simulink model "VELOCITY_MODEL"  (R2014b)
settings: Solver=ode45  StartTime=0.0  StopTime=30  RelTol=1e-3
libraries: simulink x2
settings Model: Creator=a_botros  LastModifiedBy=a_botros
settings DebuggingCC: UnderspecifiedInitializationDetection=Classic  MergeDetectMultiDrivingBlocksExec=none  StateNameClashWarn=warning

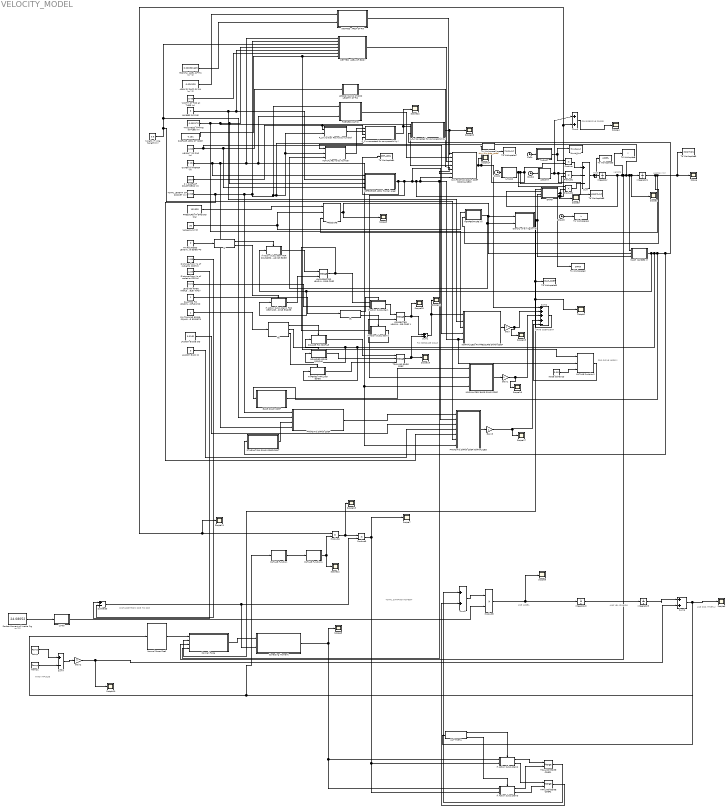
== system VELOCITY_MODEL ==
  note: FOR OGIVE NOSE!!!
  note: WIND IMPULSE
  note: ANG POS (THETA)
  note: ANG VEL (OMEGA)
  note: ANG ACCEL
  note: TOTAL DAMPING MOMENT
  note: DISTANCE FROM COG TO COP
  note: COMPRESSIVE
      | FORCE
  note: DRAG COEFICIENT
  note: FIN PRESSURE DRAG
  note: position (m)
  note: velocity
  note: accel
  1/MASS : MATLAB Function  TreatAsAtomicUnit=on
  1/MOI : MATLAB Function  TreatAsAtomicUnit=on
  ACTUAL Reynolds Number : MATLAB Function  TreatAsAtomicUnit=on
  AERODYNAMIC CHORD LENGTH OF FIN : MATLAB Function  TreatAsAtomicUnit=on
  AREA OF FACE OF FIN (m^2) : Constant  Value=0.026125
  BASE DRAG COEF : MATLAB Function  TreatAsAtomicUnit=on
  CORRECTED LEADING EDGE COEF 1 : Merge
  C_f (uncorrected for compressibility) : MATLAB Function  TreatAsAtomicUnit=on
  C_f_c (corrected for compressibility) : MATLAB Function  TreatAsAtomicUnit=on
  Clock{,1..3} (4 alike) : Clock
  Correcting Moment : MATLAB Function  TreatAsAtomicUnit=on
  DRAG : MATLAB Function  TreatAsAtomicUnit=on
  Density of air (kg/m^3) : MATLAB Function  TreatAsAtomicUnit=on
  Distance from tip of rocket to COG(m) : Constant  Value=1.88
  Distance from tip of rocket to COP(m) : Constant  Value=2.05
  FIN ROUNDED LEADING EDGE=1 RECT' LEADING EDGE =0 : Constant  Value=0
  "FIN TRAILING EDGE: SQUARE FIN PROFILE=1 ROUNDED EDGE PROFILE=2 TAPERED TRAILING EDGE=3 " : Constant
  FINENESS RATIO : MATLAB Function  TreatAsAtomicUnit=on
  FRONTAL AREA OF FIN (m^2) : Constant  Value=0.000301625
  Gain : Gain
  Gain1 : Gain
  Gain2 : Gain  Gain=0
  Gain3 : Gain
  HEIGHT OF FINS (m) : Constant  Value=0.95
  If : If  IfExpression=u1==1
  If Action Subsystem : Subsystem  TreatAsAtomicUnit=on
  If Action Subsystem FOR ROUNDED LEADING EDGE : Subsystem  TreatAsAtomicUnit=on
  If Action Subsystem1 : Subsystem  TreatAsAtomicUnit=on
  If Action Subsystem1 FOR RECTANGULAR LEADING ENDGE : Subsystem  TreatAsAtomicUnit=on
  If Action Subsystem2 : Subsystem  TreatAsAtomicUnit=on
  If Action Subsystem3 : Subsystem  TreatAsAtomicUnit=on
  If1 : If  IfExpression=u1 == 1
  If2 : If  IfExpression=u1 ==1  ElseIfExpressions=u1==2
  Integrator{,1..3} (4 alike) : Integrator
  LAUNCH GUID ID : Constant  Value=0
  LAUNCH GUIDE OD : Constant  Value=0.0161
  LEADING EDGE ANGLE (IF APPLICABLE) (RAD) : Constant  Value=0.21
  MACH NUMBER M : MATLAB Function  TreatAsAtomicUnit=on
  MATLAB Function : MATLAB Function  TreatAsAtomicUnit=on
  MATLAB Function1 : MATLAB Function  TreatAsAtomicUnit=on
  MATLAB Function2 : MATLAB Function  TreatAsAtomicUnit=on
  NORMALIZED BASE DRAG COEF : MATLAB Function  TreatAsAtomicUnit=on
  NORMALIZED FIN PRESSURE DRAG COEF : MATLAB Function  TreatAsAtomicUnit=on
  NOSE CONE CD : Constant  Value=0.05
  NUMBER OF FINS : Constant  Value=3
  Normal Force : MATLAB Function  TreatAsAtomicUnit=on
  Normal Force Coef : MATLAB Function  TreatAsAtomicUnit=on
  OUTER DIAMETER (m) : Constant  Value=0.104
  PARASITIC DRAG COEF : MATLAB Function  TreatAsAtomicUnit=on
  PARASITIC DRAG COEF NORMALIZED : MATLAB Function  TreatAsAtomicUnit=on
  PRESSURE : MATLAB Function  TreatAsAtomicUnit=on
  PRESSURE AT GROUND (Pa) : Constant  Value=101325
  Product{,1..5} (6 alike) : Product
  REFERENCE AREA (frontal area) : MATLAB Function  TreatAsAtomicUnit=on
  ROUNDED EDGE PROFILE : Subsystem  TreatAsAtomicUnit=on
  R_crit (critical Reynolds number) : MATLAB Function  TreatAsAtomicUnit=on
  R_s SURFACE ROUGHNESS (m) : Constant  Value=20E-6
  Ramp : simulink/Sources/Ramp  slope=5  start=2  X0=0
  Ramp1 : simulink/Sources/Ramp  slope=-5  start=2.0001  X0=0
  Rocket Moment of Inertia (kg m^2) : Constant  Value=24.08052
  SKN FRICTION DRAG COEF (NORMALIZED) : MATLAB Function  TreatAsAtomicUnit=on
  SLANTED FIN LEADING EDGE=1 FIN PERPENDICULAR TO AIRFLOW=0 : Constant
  SQUARE FIN PROFILE : Subsystem  TreatAsAtomicUnit=on
  STAGNATION DRAG COEFICIENT : MATLAB Function  TreatAsAtomicUnit=on
  SURFACE AREA OF NOSE : Constant  Value=0.131
  Scope{,1..22} (23 alike) : Scope
      Scope10 settings: SaveName=ScopeData10
      Scope11 settings: SaveName=ScopeData11
      Scope12 settings: SaveName=ScopeData12
      Scope13 settings: SaveName=ScopeData13
      Scope14 settings: SaveName=ScopeData14
      Scope15 settings: SaveName=ScopeData15
      Scope16 settings: SaveName=ScopeData16
      Scope17 settings: SaveName=ScopeData17
      Scope18 settings: SaveName=ScopeData18
      Scope19 settings: SaveName=ScopeData19
      Scope2 settings: SaveName=ScopeData2
      Scope20 settings: SaveName=ScopeData20
      Scope21 settings: SaveName=ScopeData21
      Scope22 settings: SaveName=ScopeData22
      Scope3 settings: SaveName=ScopeData3
      Scope4 settings: SaveName=ScopeData4
      Scope5 settings: SaveName=ScopeData5
      Scope6 settings: YMin=25000  YMax=105000  SaveName=ScopeData6
      Scope7 settings: SaveName=ScopeData7
      Scope8 settings: SaveName=ScopeData8
      Scope9 settings: SaveName=ScopeData9
  Subtract3 : Sum  Inputs=+-
  Sum : Sum  Inputs=+--
  Sum1 : Sum
  Sum2 : Sum  Inputs=++++-
  Sum3 : Sum  Inputs=|++
  Sum5 : Sum
  Sum6 : Sum  Inputs=|++
  Sum7 : Sum  Inputs=+-
  TAPERED TRAILING EDGE : Subsystem  TreatAsAtomicUnit=on
  TEMPERATURE (K) : MATLAB Function  TreatAsAtomicUnit=on
  THICKNESS OF FINS at TUBE (m) : Constant  Value=0.003175
  THRUST : MATLAB Function  TreatAsAtomicUnit=on
  TOTAL LENGTH OF ROCKET (m) : Constant  Value=2.98
  TRAILING EDGE COEF : Merge  Inputs=3
  TRAILING EDGE COEF1 : Merge
  TRAILING EDGE COEF2 : Merge
  To Workspace : ToWorkspace  VariableName=v  SampleTime=-1
  To Workspace1 : ToWorkspace  VariableName=t  SampleTime=-1
  To Workspace2 : ToWorkspace  VariableName=DRAG  SampleTime=-1
  To Workspace3 : ToWorkspace  VariableName=ACCEL  SaveFormat=Timeseries  SampleTime=-1
  To Workspace4 : ToWorkspace  VariableName=REF_AREA  SampleTime=-1
  To Workspace5 : ToWorkspace  VariableName=POSITION  SampleTime=-1
  To Workspace6 : ToWorkspace  VariableName=DRAG_COEF  SampleTime=-1
  To Workspace7 : ToWorkspace  VariableName=mass_out  SampleTime=-1
  To Workspace8 : ToWorkspace  VariableName=weight_out  SampleTime=-1
  To Workspace9 : ToWorkspace  VariableName=skin_fric_drag_cofef  SampleTime=-1
  U1+THETA : If
  "UNCORRECTED LEADING EDGE COEF " : Merge
  WEIGHT : MATLAB Function  TreatAsAtomicUnit=on
  WETTED  AREA OF BODY : MATLAB Function  TreatAsAtomicUnit=on
  WETTED  AREA OF FIN : MATLAB Function  TreatAsAtomicUnit=on
  WIDTH OF FINS at TUBE (m) : Constant  Value=0.45
  height of nose (length)(m) : Constant  Value=0.6
  t_at_ground (C) : Constant  Value=30
  "thrust_out " : ToWorkspace  VariableName=thrust_out  SampleTime=-1
  wires:
  THRUST/1(T) -> "thrust_out "/1, Product/1
  1/MASS/1(M) -> Product2/1, Product1/2, Product/2, To Workspace7/1
  Clock/1 -> THRUST/1(t)
  Clock1/1 -> 1/MASS/1(t)
  Product/1 -> Sum/1
  Clock2/1 -> WEIGHT/1(t)
  Product1/1 -> Sum/2
  DRAG/1(D) -> To Workspace2/1, Scope3/1, Scope11/1, Product4/1, Sum3/2, Product2/2
  Product2/1 -> Sum/3
  Integrator/1 -> DRAG/2(v), Normal Force/3(v), ACTUAL Reynolds Number/1(v), MACH NUMBER M/1(v), Scope1/1, Integrator1/1, To Workspace/1
  Sum/1 -> To Workspace3/1, Integrator/1
  WEIGHT/1(W) -> Sum3/1, To Workspace8/1, Product1/1
  Clock3/1 -> To Workspace1/1
  Integrator1/1 -> PRESSURE/3(x), To Workspace5/1, Scope/1, TEMPERATURE (K)/2(x)
  Density of air (kg/m^3)/1(ro) -> Normal Force/2(ro), DRAG/3(ro), MACH NUMBER M/3(ro)
  TEMPERATURE (K)/1(T) -> ACTUAL Reynolds Number/3(T), Density of air (kg/m^3)/2(T)
  t_at_ground (C)/1 -> TEMPERATURE (K)/1(t_at_ground), PRESSURE/2(t_0)
  PRESSURE/1(p) -> Density of air (kg/m^3)/1(p), MACH NUMBER M/2(p), Scope5/1
  R_s SURFACE ROUGHNESS (m)/1 -> C_f (uncorrected for compressibility)/3(R_s), R_crit (critical Reynolds number)/1(R_s)
  TOTAL LENGTH OF ROCKET (m)/1 -> PARASITIC DRAG COEF NORMALIZED/5(L), PARASITIC DRAG COEF/1(L), FINENESS RATIO/1(L), C_f (uncorrected for compressibility)/4(L), R_crit (critical Reynolds number)/2(L), ACTUAL Reynolds Number/2(L), WETTED  AREA OF BODY/2(L)
  ACTUAL Reynolds Number/1(R) -> C_f (uncorrected for compressibility)/1(R)
  R_crit (critical Reynolds number)/1(R_crit) -> C_f (uncorrected for compressibility)/2(R_crit)
  C_f (uncorrected for compressibility)/1(C_f) -> Scope22/1, C_f_c (corrected for compressibility)/1(C_f)
  MACH NUMBER M/1(M) -> If Action Subsystem1 FOR RECTANGULAR LEADING ENDGE/1(In1), If Action Subsystem FOR ROUNDED LEADING EDGE/1(In1), TAPERED TRAILING EDGE/1(In1), ROUNDED EDGE PROFILE/1(In1), SQUARE FIN PROFILE/1(In1), BASE DRAG COEF/1(M), STAGNATION DRAG COEFICIENT/1(M), C_f_c (corrected for compressibility)/2(M)
  PRESSURE AT GROUND (Pa)/1 -> PRESSURE/1(p_0)
  OUTER DIAMETER (m)/1 -> PARASITIC DRAG COEF NORMALIZED/7(OD), NORMALIZED BASE DRAG COEF/3(OD), FINENESS RATIO/2(OD), WETTED  AREA OF BODY/1(OD), PARASITIC DRAG COEF/4(OD), REFERENCE AREA (frontal area)/1(OD)
  HEIGHT OF FINS (m)/1 -> NORMALIZED FIN PRESSURE DRAG COEF/4(s), REFERENCE AREA (frontal area)/4(s), AERODYNAMIC CHORD LENGTH OF FIN/1(s)
  height of nose (length)(m)/1 -> PARASITIC DRAG COEF NORMALIZED/6(h), PARASITIC DRAG COEF/2(h), WETTED  AREA OF BODY/3(h)
  SURFACE AREA OF NOSE/1 -> WETTED  AREA OF BODY/7(A_surface_nose), MATLAB Function2/1(A)
  THICKNESS OF FINS at TUBE (m)/1 -> NORMALIZED FIN PRESSURE DRAG COEF/3(t), SKN FRICTION DRAG COEF (NORMALIZED)/4(t), REFERENCE AREA (frontal area)/3(t), WETTED  AREA OF BODY/4(t)
  NUMBER OF FINS/1 -> REFERENCE AREA (frontal area)/2(N), WETTED  AREA OF BODY/5(N), NORMALIZED FIN PRESSURE DRAG COEF/2(N)
  WIDTH OF FINS at TUBE (m)/1 -> WETTED  AREA OF BODY/6(l)
  FRONTAL AREA OF FIN (m^2)/1 -> WETTED  AREA OF FIN/2(A_front_fin)
  AREA OF FACE OF FIN (m^2)/1 -> WETTED  AREA OF FIN/1(A_face_fin)
  STAGNATION DRAG COEFICIENT/1(C_stag) -> PARASITIC DRAG COEF/3(C_stag)
  FIN ROUNDED LEADING EDGE=1 RECT' LEADING EDGE =0/1 -> If/1
  If/1 -> If Action Subsystem FOR ROUNDED LEADING EDGE/Action
  If/2 -> If Action Subsystem1 FOR RECTANGULAR LEADING ENDGE/Action
  If Action Subsystem FOR ROUNDED LEADING EDGE/1(Out1) -> "UNCORRECTED LEADING EDGE COEF "/1
  If Action Subsystem1 FOR RECTANGULAR LEADING ENDGE/1(Out1) -> "UNCORRECTED LEADING EDGE COEF "/2
  SLANTED FIN LEADING EDGE=1 FIN PERPENDICULAR TO AIRFLOW=0/1 -> If1/1
  If1/2 -> If Action Subsystem1/Action
  If1/1 -> If Action Subsystem/Action
  "UNCORRECTED LEADING EDGE COEF "/1 -> If Action Subsystem1/1(In1), If Action Subsystem/1(In1)
  LEADING EDGE ANGLE (IF APPLICABLE) (RAD)/1 -> If Action Subsystem/2(In2)
  If Action Subsystem/1(Out1) -> CORRECTED LEADING EDGE COEF 1/1
  If Action Subsystem1/1(Out1) -> CORRECTED LEADING EDGE COEF 1/2
  "FIN TRAILING EDGE: SQUARE FIN PROFILE=1 ROUNDED EDGE PROFILE=2 TAPERED TRAILING EDGE=3 "/1 -> If2/1
  If2/1 -> SQUARE FIN PROFILE/Action
  If2/2 -> ROUNDED EDGE PROFILE/Action
  If2/3 -> TAPERED TRAILING EDGE/Action
  SQUARE FIN PROFILE/1(Out1) -> TRAILING EDGE COEF/1
  ROUNDED EDGE PROFILE/1(Out1) -> TRAILING EDGE COEF/2
  TAPERED TRAILING EDGE/1(Out1) -> TRAILING EDGE COEF/3
  CORRECTED LEADING EDGE COEF 1/1 -> Scope18/1, Sum1/1
  C_f_c (corrected for compressibility)/1(C_f_c) -> Scope20/1, SKN FRICTION DRAG COEF (NORMALIZED)/1(C_f_c)
  FINENESS RATIO/1(f_b) -> SKN FRICTION DRAG COEF (NORMALIZED)/2(f_b)
  WETTED  AREA OF BODY/1(A_wet_body) -> SKN FRICTION DRAG COEF (NORMALIZED)/3(A_wet_body)
  AERODYNAMIC CHORD LENGTH OF FIN/1(c) -> SKN FRICTION DRAG COEF (NORMALIZED)/5(c)
  WETTED  AREA OF FIN/1(A_wet_fin) -> SKN FRICTION DRAG COEF (NORMALIZED)/6(A_wet_fins)
  REFERENCE AREA (frontal area)/1(A_ref) -> To Workspace4/1, Normal Force/4(A_ref), MATLAB Function2/2(A_ref), NORMALIZED FIN PRESSURE DRAG COEF/5(A_ref), SKN FRICTION DRAG COEF (NORMALIZED)/7(A_ref), DRAG/4(A_ref), PARASITIC DRAG COEF NORMALIZED/2(A_ref), NORMALIZED BASE DRAG COEF/2(A_ref)
  Sum1/1 -> Scope21/1, NORMALIZED FIN PRESSURE DRAG COEF/1(fin_pressure_drag)
  BASE DRAG COEF/1(C_base) -> NORMALIZED BASE DRAG COEF/1(C_base)
  PARASITIC DRAG COEF/1(C_parasitic) -> PARASITIC DRAG COEF NORMALIZED/1(C_parasitic)
  LAUNCH GUIDE OD/1 -> PARASITIC DRAG COEF NORMALIZED/3(r_ext)
  LAUNCH GUID ID/1 -> PARASITIC DRAG COEF NORMALIZED/4(r_int)
  TRAILING EDGE COEF/1 -> Scope19/1, Sum1/2
  SKN FRICTION DRAG COEF (NORMALIZED)/1(C_D_fric) -> Scope14/1, To Workspace9/1, Sum2/1
  Gain/1 -> Scope15/1, Sum2/2
  Gain1/1 -> Scope16/1, Sum2/3
  Gain3/1 -> Sum2/4, Scope17/1
  Sum2/1 -> Scope2/1, DRAG/1(Cd), To Workspace6/1
  Sum3/1 -> Scope4/1
  Distance from tip of rocket to COG(m)/1 -> Subtract3/2
  Distance from tip of rocket to COP(m)/1 -> Subtract3/1
  Subtract3/1 -> Product5/2, Correcting Moment/2(d_t)
  Normal Force Coef/1(C_N) -> Normal Force/1(C_N)
  Normal Force/1(N) -> Correcting Moment/1(N)
  Correcting Moment/1(M_correcting) -> If Action Subsystem3/1(N), If Action Subsystem2/1(N), Scope8/1
  Sum5/1 -> Product3/1
  Rocket Moment of Inertia (kg m^2)/1 -> 1/MOI/1(u)
  1/MOI/1(y) -> Product3/2
  Product3/1 -> Scope9/1, Integrator2/1
  Integrator2/1 -> Integrator3/1
  Gain2/1 -> Scope10/1, Sum6/2
  Integrator3/1 -> Sum6/1
  Sum6/1 -> U1+THETA/1, Scope6/1, MATLAB Function/1(deg), Normal Force Coef/1(theta)
  Ramp/1 -> Sum7/1
  Ramp1/1 -> Sum7/2
  Sum7/1 -> Gain2/1
  MATLAB Function/1(rad) -> MATLAB Function1/1(u)
  MATLAB Function1/1(y) -> Product4/2, Scope12/1
  Product4/1 -> Scope13/1, Product5/1
  Product5/1 -> If Action Subsystem3/2(D), If Action Subsystem2/2(D), Scope7/1
  U1+THETA/1 -> If Action Subsystem2/Action
  U1+THETA/2 -> If Action Subsystem3/Action
  If Action Subsystem2/1(Nout) -> TRAILING EDGE COEF1/1
  If Action Subsystem3/1(Nout) -> TRAILING EDGE COEF1/2
  If Action Subsystem3/2(Dout) -> TRAILING EDGE COEF2/2
  If Action Subsystem2/2(Dout) -> TRAILING EDGE COEF2/1
  TRAILING EDGE COEF1/1 -> Sum5/1
  TRAILING EDGE COEF2/1 -> Sum5/2
  NORMALIZED FIN PRESSURE DRAG COEF/1(C_D_pressure) -> Gain/1
  NORMALIZED BASE DRAG COEF/1(C_base_n) -> Gain1/1
  PARASITIC DRAG COEF NORMALIZED/1(C_parasitic_norm) -> Gain3/1
  NOSE CONE CD/1 -> MATLAB Function2/3(CND)
  MATLAB Function2/1(y) -> Sum2/5

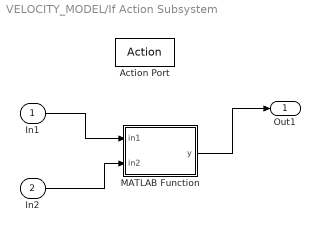
== system VELOCITY_MODEL/If Action Subsystem ==
  In1 : Inport
  In2 : Inport  Port=2
  Action Port : ActionPort  ActionType=then
  MATLAB Function : MATLAB Function  TreatAsAtomicUnit=on
  Out1 : Outport
  wires:
  In1/1 -> MATLAB Function/1(in1)
  In2/1 -> MATLAB Function/2(in2)
  MATLAB Function/1(y) -> Out1/1

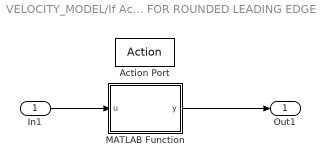
== system VELOCITY_MODEL/If Action Subsystem FOR ROUNDED LEADING EDGE ==
  In1 : Inport
  Action Port : ActionPort  ActionType=then
  MATLAB Function : MATLAB Function  TreatAsAtomicUnit=on
  Out1 : Outport
  wires:
  In1/1 -> MATLAB Function/1(u)
  MATLAB Function/1(y) -> Out1/1

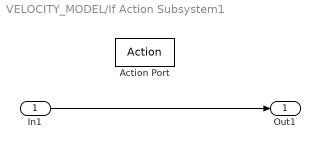
== system VELOCITY_MODEL/If Action Subsystem1 ==
  In1 : Inport
  Action Port : ActionPort  ActionType=else
  Out1 : Outport
  wires:
  In1/1 -> Out1/1

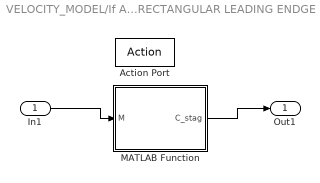
== system VELOCITY_MODEL/If Action Subsystem1 FOR RECTANGULAR LEADING ENDGE ==
  In1 : Inport
  Action Port : ActionPort  ActionType=else
  MATLAB Function : MATLAB Function  TreatAsAtomicUnit=on
  Out1 : Outport
  wires:
  In1/1 -> MATLAB Function/1(M)
  MATLAB Function/1(C_stag) -> Out1/1

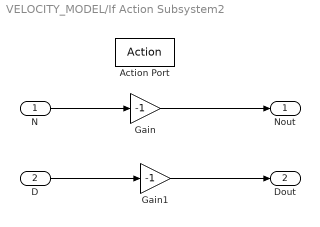
== system VELOCITY_MODEL/If Action Subsystem2 ==
  N : Inport
  D : Inport  Port=2
  Action Port : ActionPort  ActionType=then
  Gain : Gain  Gain=-1
  Gain1 : Gain  Gain=-1
  Nout : Outport
  Dout : Outport  Port=2
  wires:
  N/1 -> Gain/1
  Gain/1 -> Nout/1
  D/1 -> Gain1/1
  Gain1/1 -> Dout/1

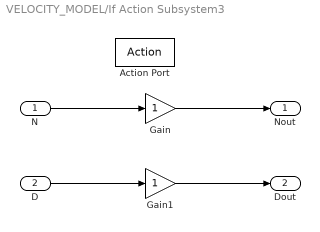
== system VELOCITY_MODEL/If Action Subsystem3 ==
  N : Inport
  D : Inport  Port=2
  Action Port : ActionPort  ActionType=else
  Gain : Gain
  Gain1 : Gain
  Nout : Outport
  Dout : Outport  Port=2
  wires:
  N/1 -> Gain/1
  Gain/1 -> Nout/1
  D/1 -> Gain1/1
  Gain1/1 -> Dout/1

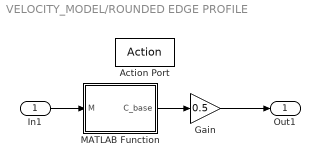
== system VELOCITY_MODEL/ROUNDED EDGE PROFILE ==
  In1 : Inport
  Action Port : ActionPort  ActionType=elseif
  Gain : Gain  Gain=0.5
  MATLAB Function : MATLAB Function  TreatAsAtomicUnit=on
  Out1 : Outport
  wires:
  In1/1 -> MATLAB Function/1(M)
  MATLAB Function/1(C_base) -> Gain/1
  Gain/1 -> Out1/1

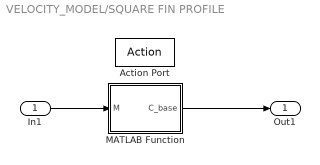
== system VELOCITY_MODEL/SQUARE FIN PROFILE ==
  In1 : Inport
  Action Port : ActionPort  ActionType=then
  MATLAB Function : MATLAB Function  TreatAsAtomicUnit=on
  Out1 : Outport
  wires:
  In1/1 -> MATLAB Function/1(M)
  MATLAB Function/1(C_base) -> Out1/1

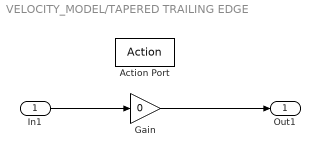
== system VELOCITY_MODEL/TAPERED TRAILING EDGE ==
  In1 : Inport
  Action Port : ActionPort  ActionType=else
  Gain : Gain  Gain=0
  Out1 : Outport
  wires:
  In1/1 -> Gain/1
  Gain/1 -> Out1/1

== matlab function VELOCITY_MODEL/WEIGHT ==
  data: t input; W output
function W   = WEIGHT( t )
if t<=4.7012
    W=(75.94*t^2-1234.5*t+20937)/1000*9.80665 

else
    W=17092/1000*9.80665 
end


end

== matlab function VELOCITY_MODEL/THRUST ==
  data: t input; T output
function  T  = THRUST(t)
%YIELDS THRUST CURVE OVER TIME
if t<0.08
    T=4000000*t^3-462933*t^2+41915*t+209.66
elseif t<0.15935
    T=-4701*t+2748.7
elseif t<0.21276 
    T=-1133.2*t+2223.6 
elseif t<0.32775
    T=787.15*t+1850.2
elseif t<0.57775
    T=-754.4*t+2339.9  
elseif t<0.72775
    T=-251*t+2070.7 
elseif t<1.7277
    T=-70.147*t+1947.4
elseif t<3.3777
    T=-31.421*t^2-9.1503*t+1930.8
elseif t<3.9777
    T=3656.6*t^3-39167*t^2+137806*t-158018
elseif t<4.5277
    T=-1051.8*t+4709.4
else
    T=0
    
      
   end


end

== matlab function VELOCITY_MODEL/1//MASS ==
  data: t input; M output
function M   = MASSRECIP( t )

if t<=4.7012
    M=1/((75.94*t^2-1234.5*t+20937)/1000)

else
    M=1/(17092/1000) 
end

end

== matlab function VELOCITY_MODEL/DRAG ==
  data: Cd input; D output; v input; ro input; A_ref input
function D = DRAG(Cd, v, ro, A_ref)
%#codegen
D=0.5*Cd*v^2*A_ref*ro
end

== matlab function VELOCITY_MODEL/NORMALIZED FIN PRESSURE DRAG COEF ==
  data: fin_pressure_drag input; C_D_pressure output; N input; t input; s input; A_ref input
function C_D_pressure = PRESS(fin_pressure_drag, N ,t ,s, A_ref)
%#codegen

C_D_pressure = fin_pressure_drag*N*t*s/A_ref;
end

== matlab function VELOCITY_MODEL/Density of air (kg//m^3) ==
  data: p input; ro output; T input
function ro = DENSITYOFAIR(p,T)
%#codegen
ro=p*0.0289644/(8.31447*T)
end

== matlab function VELOCITY_MODEL/TEMPERATURE (K) ==
  data: t_at_ground input; T output; x input
function T = t(t_at_ground, x)
%#codegen
double m;
if x<11000
    m=-6.5
elseif x<11019
    m=0
else 
    m=1
end
    
    
    
    
    
T=(t_at_ground+274.15-m/1000*x)
end

== matlab function VELOCITY_MODEL/If Action Subsystem/MATLAB Function ==
  data: in1 input; y output; in2 input
function y = fcn(in1, in2)
%#codegen
y=in1*cos(in2)^2
end

== matlab function VELOCITY_MODEL/REFERENCE AREA (frontal area) ==
  data: OD input; A_ref output; N input; t input; s input
function A_ref = REFAREA(OD, N, t, s)
%#codegen

%A_ref=3.14159*OD^2/4+t*s*N
A_ref=0.0084949
end

== matlab function VELOCITY_MODEL/BASE DRAG COEF ==
  data: M input; C_base output
function C_base = BASEDRAG(M)
%#codegen
if M<1
    C_base=0.12+0.13*M^2
else
    C_base=0.25/M
end

end

== matlab function VELOCITY_MODEL/PARASITIC DRAG COEF ==
  data: L input; C_parasitic output; h input; C_stag input; OD input
function C_parasitic = PARASITICDRAG(L,h,C_stag,OD)
%#codegen
C_parasitic=max(1.3-0.3*(L-h)/OD, 1)*C_stag
end

== matlab function VELOCITY_MODEL/R_crit (critical Reynolds number) ==
  data: R_s input; R_crit output; L input
function R_crit = CRITREN(R_s, L)
%#codegen

R_crit=51*(R_s/L)^(-1.039);
end

== matlab function VELOCITY_MODEL/C_f (uncorrected for compressibility) ==
  data: R input; C_f output; R_crit input; R_s input; L input
function C_f = SKNDRAGCOEF(R, R_crit, R_s, L)
%#codegen
if R<1E4
  C_f=0.0148
elseif R<R_crit
  C_f=1/(1.5*log(R)-5.6)^2 
else
  C_f=0.032*(R_s/L)^(0.2)
end 


end

== matlab function VELOCITY_MODEL/ACTUAL Reynolds Number ==
  data: v input; R output; L input; T input
function R = ACTREN(v, L, T)
%#codegen

R=v*L/(-1E-14*T^3+1E-10*T^2+3E-8*T-3E-6);
end

== matlab function VELOCITY_MODEL/MACH NUMBER M ==
  data: v input; M output; p input; ro input
function M = MACH(v, p, ro)
%#codegen

M=v/sqrt(1.4*p/ro)
end

== matlab function VELOCITY_MODEL/C_f_c (corrected for compressibility) ==
  data: C_f input; C_f_c output; M input
function C_f_c = SKNDRAGCOEFCORR(C_f, M)
%#codegen
double CC;
CC=C_f*(1-0.1*M^2);

if CC>C_f
  C_f_c=CC
else
  C_f_c=C_f
end

end

== matlab function VELOCITY_MODEL/PRESSURE ==
  data: p_0 input; p output; t_0 input; x input
function p = PRESSURE(p_0, t_0, x)
%#codegen
p=p_0*(1-0.0065*x/(t_0+274.15))^(9.80665*0.0289644/(8.31447*0.0065))
end

== matlab function VELOCITY_MODEL/FINENESS RATIO ==
  data: L input; f_b output; OD input
function f_b = FINENESS(L, OD)
%#codegen

f_b=L/OD
end

== matlab function VELOCITY_MODEL/AERODYNAMIC CHORD LENGTH OF FIN ==
  data: s input; c output
function c = ACL(s)
%#codegen
c=s
end

== matlab function VELOCITY_MODEL/SKN FRICTION DRAG COEF (NORMALIZED) ==
  data: C_f_c input; C_D_fric output; f_b input; A_wet_body input; t input; c input; A_wet_fins input; A_ref input
function C_D_fric = fcn(C_f_c, f_b, A_wet_body, t, c, A_wet_fins, A_ref)
%#codegen
C_D_fric=C_f_c*( (1+1/(2*f_b))*A_wet_body + (1+2*t/c)*A_wet_fins  )/A_ref
end

== matlab function VELOCITY_MODEL/WETTED  AREA OF BODY ==
  data: OD input; A_wet_body output; L input; h input; t input; N input; l input; A_surface_nose input
function A_wet_body = WAB(OD, L, h, t, N, l, A_surface_nose)
%#codegen
A_wet_body=3.14159*OD*(L-h)+A_surface_nose-t*l*N
end

== matlab function VELOCITY_MODEL/WETTED  AREA OF FIN ==
  data: A_face_fin input; A_wet_fin output; A_front_fin input
function A_wet_fin = AWF(A_face_fin, A_front_fin)
%#codegen
A_wet_fin=2*A_face_fin+A_front_fin
end

== matlab function VELOCITY_MODEL/NORMALIZED BASE DRAG COEF ==
  data: C_base input; C_base_n output; A_ref input; OD input
function C_base_n = NORMBASEDRAG(C_base, A_ref, OD)
%#codegen

C_base_n=C_base*3.14159*(OD^2/4)/A_ref
end

== matlab function VELOCITY_MODEL/SQUARE FIN PROFILE/MATLAB Function ==
  data: M input; C_base output
function C_base = BASEDRAG(M)
%#codegen
if M<1
    C_base=0.12+0.13*M^2
else
    C_base=0.25/M
end

end

== matlab function VELOCITY_MODEL/STAGNATION DRAG COEFICIENT ==
  data: M input; C_stag output
function C_stag = STAGDRAGCOEF(M)
%#codegen
if M<1
    C_stag=0.85*(1+M^2/4+M^4/40)
else
    C_stag=0.85*(1.84-0.76/M^2+0.166/M^4+0.035/M^6)
end

end

== matlab function VELOCITY_MODEL/If Action Subsystem FOR ROUNDED LEADING EDGE/MATLAB Function ==
  data: u input; y output
function y = fcn(u)
%#codegen
if u<0.9
    y=(1-u^2)^(-0.417)-1
elseif u<1
    y=1-1.785*(u-0.9)
else
    y=1.214-0.502/u^2+0.1095/u^4
end
end

== matlab function VELOCITY_MODEL/If Action Subsystem1 FOR RECTANGULAR LEADING ENDGE/MATLAB Function ==
  data: M input; C_stag output
function C_stag = STAGDRAGCOEF(M)
%#codegen
if M<1
    C_stag=0.85*(1+M^2/4+M^4/40)
else
    C_stag=0.85*(1.84-0.76/M^2+0.166/M^4+0.035/M^6)
end

end

== matlab function VELOCITY_MODEL/ROUNDED EDGE PROFILE/MATLAB Function ==
  data: M input; C_base output
function C_base = BASEDRAG(M)
%#codegen
if M<1
    C_base=0.12+0.13*M^2
else
    C_base=0.25/M
end

end

== matlab function VELOCITY_MODEL/PARASITIC DRAG COEF NORMALIZED ==
  data: C_parasitic input; C_parasitic_norm output; A_ref input; r_ext input; r_int input; L input; h input; OD input
function C_parasitic_norm = fcn(C_parasitic, A_ref, r_ext, r_int, L, h, OD)
%#codegen

C_parasitic_norm=C_parasitic*(3.14159*(r_ext^2-r_int^2)*max(1-(L-h)/OD, 0))/A_ref

== matlab function VELOCITY_MODEL/MATLAB Function ==
  data: deg input; rad output
function rad = fcn(deg)
%#codegen

rad = deg*3.141592652/180;
end

== matlab function VELOCITY_MODEL/MATLAB Function1 ==
  data: u input; y output
function y = s_i_n(u)
%#codegen

y = sin(u);

== matlab function VELOCITY_MODEL/MATLAB Function2 ==
  data: A input; y output; A_ref input; CND input
function y = fcn(A, A_ref, CND)
%#codegen

y = CND*A/A_ref;

== matlab function VELOCITY_MODEL/Correcting Moment ==
  data: N input; M_correcting output; d_t input
function M_correcting = CRCTNGMMNT(N,d_t)
%#codegen

M_correcting=N*d_t;
end

== matlab function VELOCITY_MODEL/Normal Force ==
  data: C_N input; N output; ro input; v input; A_ref input
function N = NRMLFRCE(C_N, ro, v, A_ref)
%#codegen

N=C_N*0.5*ro*v^2*A_ref;
end

== matlab function VELOCITY_MODEL/Normal Force Coef ==
  data: theta input; C_N output
function C_N = NRMLFRCECOEF(theta)
%#codegen

C_N=-0.0001*theta^3+0.0125*theta^2+0.2091*theta;
end

== matlab function VELOCITY_MODEL/1//MOI ==
  data: u input; y output
function y = fcn(u)
%#codegen

y = 1/u;
